simulink model "even_and_odd"  (R2017b)
settings: Solver=FixedStepDiscrete  StartTime=0.0  StopTime=10.0  RelTol=1e-3
settings Model: Creator=ibrahim  LastModifiedBy=ibrahim
settings OptimizationCC: DefaultParameterBehavior=Inlined  PassReuseOutputArgsAs=Individual arguments
settings DebuggingCC: ParameterTunabilityLossMsg=error
settings SFSimCC: MATLABDynamicMemAlloc=off
settings RTWCC: SystemTargetFile=ert.tlc  GenCodeOnly=on  TemplateMakefile=ert_default_tmf  GenerateReport=on  IncludeHyperlinkInReport=on  LaunchReport=on  GenerateTraceInfo=on  GenerateTraceReport=on  GenerateTraceReportSl=on  GenerateTraceReportSf=on  GenerateTraceReportEml=on  GenerateWebview=on
settings CodeAppCC: ForceParamTrailComments=on  IgnoreCustomStorageClasses=off  OperatorAnnotations=on  SimulinkDataObjDesc=on  SFDataObjDesc=on  InsertBlockDesc=on
settings ERTTargetCC: TargetLangStandard=C99 (ISO)  GenerateSampleERTMain=on  InlinedParameterPlacement=NonHierarchical  ERTCustomFileTemplate=example_file_process.tlc

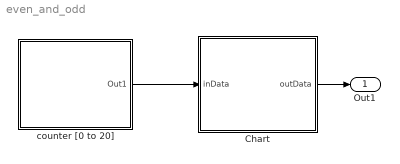
== system even_and_odd ==
  Chart : Stateflow chart  TreatAsAtomicUnit=on
  counter [0 to 20] : Subsystem
  Out1 : Outport
  wires:
  counter [0 to 20]/1(Out1) -> Chart/1(inData)
  Chart/1(outData) -> Out1/1

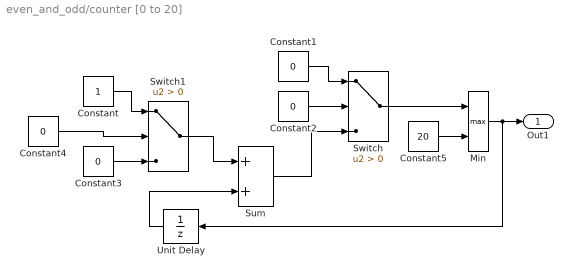
== system even_and_odd/counter [0 to 20] ==
  Constant : Constant
  Constant{1..4} (4 alike) : Constant  Value=0
  Constant5 : Constant  Value=20
  Min : MinMax  Function=max  Inputs=2
  Sum : Sum
  Switch : Switch  Criteria=u2 > Threshold
  Switch1 : Switch  Criteria=u2 > Threshold
  Unit Delay : UnitDelay  SampleTime=-1
  Out1 : Outport
  wires:
  Switch1/1 -> Sum/1
  Unit Delay/1 -> Sum/2
  Switch/1 -> Min/1
  Constant5/1 -> Min/2
  Min/1 -> Out1/1, Unit Delay/1
  Constant/1 -> Switch1/1
  Constant1/1 -> Switch/1
  Constant4/1 -> Switch1/2
  Constant2/1 -> Switch/2
  Sum/1 -> Switch/3
  Constant3/1 -> Switch1/3

== stateflow chart even_and_odd/Chart ==
  state odd
    entry:
    outData = 1;
    exit:
    outData = 0;
  state even
    entry:
    outData = 1;
    exit:
    outData = 0;
  (default) -> even
  even -> odd : [(inData & 1 == 1)]
  odd -> even : [(inData & 1 == 0)]
  data: inData input; outData output
